simulink model "continuous_model"  (R2023b)
settings: Solver=VariableStepAuto  StartTime=0.0  StopTime=t_fin  RelTol=1e-3
values from neighbouring files (symbols this model uses):
  a0 = 0.00376903    [model_setup.m]
  a1 = 0.0731193    [model_setup.m]
  a2 = 0.469961    [model_setup.m]
  alpha1 = 0.42    [model_setup.m]
  alpha2 = 0.19    [model_setup.m]
  alpha3 = 1.5    [model_setup.m]
  alpha4 = 0.95    [model_setup.m]
  b0 = 0.0050882    [model_setup.m]
  u_max = u_maxs(i)    [ex6.m]    (also in ex8.m = 0.5; model_setup.m = 1)
  u_min = 0    [ex6.m]    (also in ex8.m; model_setup.m)
  u_step_time = 10    [model_setup.m]
settings Model: Creator=vistek528  LastModifiedBy=vistek528
settings DataIOCC: ReturnWorkspaceOutputs=off

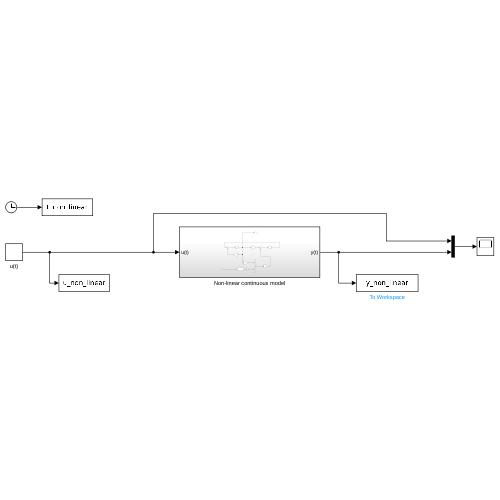
[thumbnail: Simulink's stored preview of the top-level diagram]
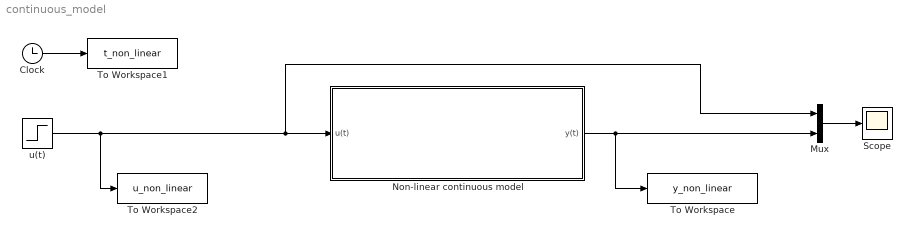
== system continuous_model ==
  Clock : Clock
  Mux : Mux  Inputs=2
  Non-linear continuous model : Subsystem
  Scope : Scope
  To Workspace : ToWorkspace  VariableName=y_non_linear  SaveFormat=Timeseries  SampleTime=-1
  To Workspace1 : ToWorkspace  VariableName=t_non_linear  SaveFormat=Timeseries  SampleTime=-1
  To Workspace2 : ToWorkspace  VariableName=u_non_linear  SaveFormat=Timeseries  SampleTime=-1
  u(t) : Step  Time=u_step_time  Before=u_min  After=u_max  SampleTime=0
  wires:
  Clock/1 -> To Workspace1/1
  u(t)/1 -> To Workspace2/1, Mux/1, Non-linear continuous model/1(u(t))
  Non-linear continuous model/1(y(t)) -> To Workspace/1, Mux/2
  Mux/1 -> Scope/1

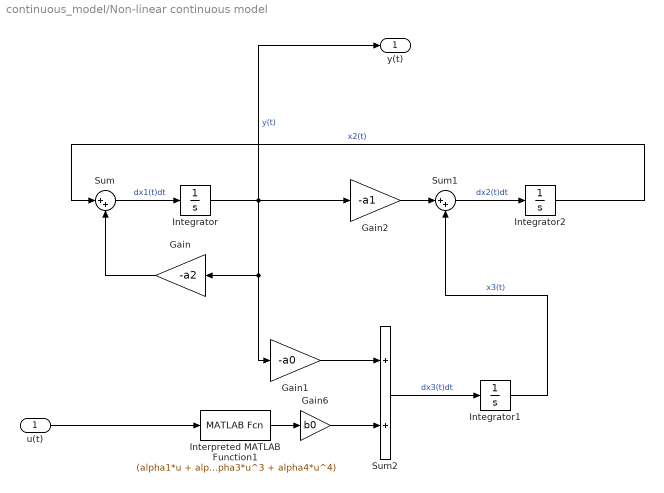
== system continuous_model/Non-linear continuous model ==
  u(t) : Inport
  Gain : Gain  Gain=-a2
  Gain1 : Gain  Gain=-a0
  Gain2 : Gain  Gain=-a1
  Gain6 : Gain  Gain=b0
  Integrator : Integrator
  Integrator1 : Integrator
  Integrator2 : Integrator
  Interpreted MATLAB Function1 : MATLABFcn  MATLABFcn=(alpha1*u + alpha2*u^2 + alpha3*u^3 + alpha4*u^4)
  Sum : Sum  Inputs=|++
  Sum1 : Sum  Inputs=|++
  Sum2 : Sum
  y(t) : Outport
  wires:
  Interpreted MATLAB Function1/1 -> Gain6/1
  Gain6/1 -> Sum2/2
  Sum2/1 -> Integrator1/1  "dx3(t)dt"
  Integrator1/1 -> Sum1/2  "x3(t)"
  Gain/1 -> Sum/2
  Sum1/1 -> Integrator2/1  "dx2(t)dt"
  Gain2/1 -> Sum1/1
  Integrator2/1 -> Sum/1  "x2(t)"
  Gain1/1 -> Sum2/1
  Sum/1 -> Integrator/1  "dx1(t)dt"
  Integrator/1 -> y(t)/1, Gain2/1, Gain1/1, Gain/1  "y(t)"
  u(t)/1 -> Interpreted MATLAB Function1/1
